simulink model "model"  (R2014a)
settings: Solver=VariableStepAuto  StartTime=0.0  StopTime=10.0  RelTol=1e-3
libraries: powerlib x73
settings Model: Creator=lej  LastModifiedBy=leimhofe
settings DataIOCC: SaveFormat=Dataset
settings OptimizationCC: SimCompilerOptimization=off
settings DebuggingCC: MergeDetectMultiDrivingBlocksExec=error  SolverPrmCheckMsg=none  FrameProcessingCompatibilityMsg=error  AllowSymbolicDim=off
settings HardwareCC: ProdBitPerPointer=64  ProdLargestAtomicFloat=Float  ProdIntDivRoundTo=Zero  ProdEndianess=LittleEndian  ProdWordSize=64  ProdHWDeviceType=Intel->x86-64 (Windows64)
settings RTWCC: RTWCompilerOptimization=off
settings GRTTargetCC: GeneratePreprocessorConditionals=Use local settings
settings ConfigComp: CovMetricSettings=dw  CovHtmlReporting=on  CovSaveCumulativeToWorkspaceVar=on  CovSaveSingleToWorkspaceVar=on  CovExternalEMLEnable=off

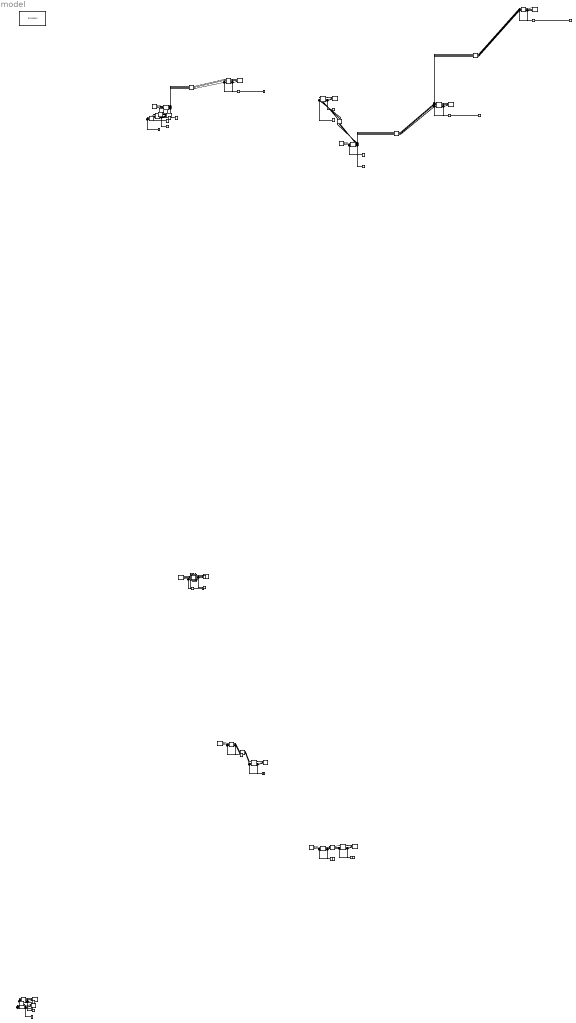
== system model ==
  note: 220000 Volts Power Line
  G_329137671_Termoeléctrica_Cospique : powerlib/Electrical Sources/Three-Phase Source  Voltage=220000  PhaseAngle=0  Frequency=60  InternalConnection=Yg  SpecifyImpedance=on  Resistance=0.8929  Inductance=16.58e-3  ShortCircuitLevel=100e6  BaseVoltage=220000  XRratio=7  BusType=swing  Pref=0  Qref=0  Qmin=-inf  Qmax=inf
  L_{42527718,88597989,108961999,133889140,169000716,169248620,235350409,265884598..265884599,329111639,329112852,329137670,329323507,330857322,331119341} (15 alike) : powerlib/Elements/Three-Phase Series RLC Load  LConnTagsString=A|B|C  Configuration=Y (grounded)  NominalVoltage=220000  NominalFrequency=60  ActivePower=100000  InductivePower=100  CapacitivePower=100  Measurements=None  LoadType=constant Z
  T_108961999__ : powerlib/Elements/Three-Phase Transformer (Two Windings)  Winding1Connection=Yg  UNITS=pu  NominalPower=[ 250e6 , 60 ]  Winding1=[220000,0.002,0.08]  Winding2Connection=Yg  Winding2=[220000,0.002,0.08]  SetSaturation=off  Rm=500  Lm=500  Saturation=[ 0,0 ; 0.0024,1.2 ; 1.0,1.52 ]  Hysteresis=off  DataFile='hysteresis'  SetInitialFlux=off  InitialFluxes=[ 0.8 , -0.8 , 0.7 ]  Measurements=None  MoreParameters=off  BreakLoop=off  DataType=off  TransfoNumber=1
  T_133889140__Ternera : powerlib/Elements/Three-Phase Transformer (Two Windings)  Winding1Connection=Yg  UNITS=pu  NominalPower=[ 250e6 , 60 ]  Winding1=[220000,0.002,0.08]  Winding2Connection=Yg  Winding2=[220000,0.002,0.08]  SetSaturation=off  Rm=500  Lm=500  Saturation=[ 0,0 ; 0.0024,1.2 ; 1.0,1.52 ]  Hysteresis=off  DataFile='hysteresis'  SetInitialFlux=off  InitialFluxes=[ 0.8 , -0.8 , 0.7 ]  Measurements=None  MoreParameters=off  BreakLoop=off  DataType=off  TransfoNumber=1
  T_169000716__ : powerlib/Elements/Three-Phase Transformer (Two Windings)  Winding1Connection=Yg  UNITS=pu  NominalPower=[ 250e6 , 60 ]  Winding1=[220000,0.002,0.08]  Winding2Connection=Yg  Winding2=[220000,0.002,0.08]  SetSaturation=off  Rm=500  Lm=500  Saturation=[ 0,0 ; 0.0024,1.2 ; 1.0,1.52 ]  Hysteresis=off  DataFile='hysteresis'  SetInitialFlux=off  InitialFluxes=[ 0.8 , -0.8 , 0.7 ]  Measurements=None  MoreParameters=off  BreakLoop=off  DataType=off  TransfoNumber=1
  T_169248620_220000_ : powerlib/Elements/Three-Phase Transformer (Two Windings)  Winding1Connection=Yg  UNITS=pu  NominalPower=[ 250e6 , 60 ]  Winding1=[220000,0.002,0.08]  Winding2Connection=Yg  Winding2=[220000,0.002,0.08]  SetSaturation=off  Rm=500  Lm=500  Saturation=[ 0,0 ; 0.0024,1.2 ; 1.0,1.52 ]  Hysteresis=off  DataFile='hysteresis'  SetInitialFlux=off  InitialFluxes=[ 0.8 , -0.8 , 0.7 ]  Measurements=None  MoreParameters=off  BreakLoop=off  DataType=off  TransfoNumber=1
  T_235350409__ : powerlib/Elements/Three-Phase Transformer (Two Windings)  Winding1Connection=Yg  UNITS=pu  NominalPower=[ 250e6 , 60 ]  Winding1=[220000,0.002,0.08]  Winding2Connection=Yg  Winding2=[220000,0.002,0.08]  SetSaturation=off  Rm=500  Lm=500  Saturation=[ 0,0 ; 0.0024,1.2 ; 1.0,1.52 ]  Hysteresis=off  DataFile='hysteresis'  SetInitialFlux=off  InitialFluxes=[ 0.8 , -0.8 , 0.7 ]  Measurements=None  MoreParameters=off  BreakLoop=off  DataType=off  TransfoNumber=1
  T_265884598__ : powerlib/Elements/Three-Phase Transformer (Two Windings)  Winding1Connection=Yg  UNITS=pu  NominalPower=[ 250e6 , 60 ]  Winding1=[220000,0.002,0.08]  Winding2Connection=Yg  Winding2=[220000,0.002,0.08]  SetSaturation=off  Rm=500  Lm=500  Saturation=[ 0,0 ; 0.0024,1.2 ; 1.0,1.52 ]  Hysteresis=off  DataFile='hysteresis'  SetInitialFlux=off  InitialFluxes=[ 0.8 , -0.8 , 0.7 ]  Measurements=None  MoreParameters=off  BreakLoop=off  DataType=off  TransfoNumber=1
  T_265884599__ : powerlib/Elements/Three-Phase Transformer (Two Windings)  Winding1Connection=Yg  UNITS=pu  NominalPower=[ 250e6 , 60 ]  Winding1=[220000,0.002,0.08]  Winding2Connection=Yg  Winding2=[220000,0.002,0.08]  SetSaturation=off  Rm=500  Lm=500  Saturation=[ 0,0 ; 0.0024,1.2 ; 1.0,1.52 ]  Hysteresis=off  DataFile='hysteresis'  SetInitialFlux=off  InitialFluxes=[ 0.8 , -0.8 , 0.7 ]  Measurements=None  MoreParameters=off  BreakLoop=off  DataType=off  TransfoNumber=1
  T_329111639_220000_ : powerlib/Elements/Three-Phase Transformer (Two Windings)  Winding1Connection=Yg  UNITS=pu  NominalPower=[ 250e6 , 60 ]  Winding1=[220000,0.002,0.08]  Winding2Connection=Yg  Winding2=[220000,0.002,0.08]  SetSaturation=off  Rm=500  Lm=500  Saturation=[ 0,0 ; 0.0024,1.2 ; 1.0,1.52 ]  Hysteresis=off  DataFile='hysteresis'  SetInitialFlux=off  InitialFluxes=[ 0.8 , -0.8 , 0.7 ]  Measurements=None  MoreParameters=off  BreakLoop=off  DataType=off  TransfoNumber=1
  T_329112852__ : powerlib/Elements/Three-Phase Transformer (Two Windings)  Winding1Connection=Yg  UNITS=pu  NominalPower=[ 250e6 , 60 ]  Winding1=[220000,0.002,0.08]  Winding2Connection=Yg  Winding2=[220000,0.002,0.08]  SetSaturation=off  Rm=500  Lm=500  Saturation=[ 0,0 ; 0.0024,1.2 ; 1.0,1.52 ]  Hysteresis=off  DataFile='hysteresis'  SetInitialFlux=off  InitialFluxes=[ 0.8 , -0.8 , 0.7 ]  Measurements=None  MoreParameters=off  BreakLoop=off  DataType=off  TransfoNumber=1
  T_329137670__ : powerlib/Elements/Three-Phase Transformer (Two Windings)  Winding1Connection=Yg  UNITS=pu  NominalPower=[ 250e6 , 60 ]  Winding1=[220000,0.002,0.08]  Winding2Connection=Yg  Winding2=[220000,0.002,0.08]  SetSaturation=off  Rm=500  Lm=500  Saturation=[ 0,0 ; 0.0024,1.2 ; 1.0,1.52 ]  Hysteresis=off  DataFile='hysteresis'  SetInitialFlux=off  InitialFluxes=[ 0.8 , -0.8 , 0.7 ]  Measurements=None  MoreParameters=off  BreakLoop=off  DataType=off  TransfoNumber=1
  T_329323507__ : powerlib/Elements/Three-Phase Transformer (Two Windings)  Winding1Connection=Yg  UNITS=pu  NominalPower=[ 250e6 , 60 ]  Winding1=[220000,0.002,0.08]  Winding2Connection=Yg  Winding2=[220000,0.002,0.08]  SetSaturation=off  Rm=500  Lm=500  Saturation=[ 0,0 ; 0.0024,1.2 ; 1.0,1.52 ]  Hysteresis=off  DataFile='hysteresis'  SetInitialFlux=off  InitialFluxes=[ 0.8 , -0.8 , 0.7 ]  Measurements=None  MoreParameters=off  BreakLoop=off  DataType=off  TransfoNumber=1
  T_330857322__ : powerlib/Elements/Three-Phase Transformer (Two Windings)  Winding1Connection=Yg  UNITS=pu  NominalPower=[ 250e6 , 60 ]  Winding1=[220000,0.002,0.08]  Winding2Connection=Yg  Winding2=[220000,0.002,0.08]  SetSaturation=off  Rm=500  Lm=500  Saturation=[ 0,0 ; 0.0024,1.2 ; 1.0,1.52 ]  Hysteresis=off  DataFile='hysteresis'  SetInitialFlux=off  InitialFluxes=[ 0.8 , -0.8 , 0.7 ]  Measurements=None  MoreParameters=off  BreakLoop=off  DataType=off  TransfoNumber=1
  T_331119341__ : powerlib/Elements/Three-Phase Transformer (Two Windings)  Winding1Connection=Yg  UNITS=pu  NominalPower=[ 250e6 , 60 ]  Winding1=[220000,0.002,0.08]  Winding2Connection=Yg  Winding2=[220000,0.002,0.08]  SetSaturation=off  Rm=500  Lm=500  Saturation=[ 0,0 ; 0.0024,1.2 ; 1.0,1.52 ]  Hysteresis=off  DataFile='hysteresis'  SetInitialFlux=off  InitialFluxes=[ 0.8 , -0.8 , 0.7 ]  Measurements=None  MoreParameters=off  BreakLoop=off  DataType=off  TransfoNumber=1
  T_42527718__Central_electrica_Torca : powerlib/Elements/Three-Phase Transformer (Two Windings)  Winding1Connection=Yg  UNITS=pu  NominalPower=[ 250e6 , 60 ]  Winding1=[220000,0.002,0.08]  Winding2Connection=Yg  Winding2=[220000,0.002,0.08]  SetSaturation=off  Rm=500  Lm=500  Saturation=[ 0,0 ; 0.0024,1.2 ; 1.0,1.52 ]  Hysteresis=off  DataFile='hysteresis'  SetInitialFlux=off  InitialFluxes=[ 0.8 , -0.8 , 0.7 ]  Measurements=None  MoreParameters=off  BreakLoop=off  DataType=off  TransfoNumber=1
  T_88597989__Sabanalarga : powerlib/Elements/Three-Phase Transformer (Two Windings)  Winding1Connection=Yg  UNITS=pu  NominalPower=[ 250e6 , 60 ]  Winding1=[220000,0.002,0.08]  Winding2Connection=Yg  Winding2=[220000,0.002,0.08]  SetSaturation=off  Rm=500  Lm=500  Saturation=[ 0,0 ; 0.0024,1.2 ; 1.0,1.52 ]  Hysteresis=off  DataFile='hysteresis'  SetInitialFlux=off  InitialFluxes=[ 0.8 , -0.8 , 0.7 ]  Measurements=None  MoreParameters=off  BreakLoop=off  DataType=off  TransfoNumber=1
  _CN_108961999_220000_CN_133889140_220000 : powerlib/Elements/Distributed Parameters Line  Phases=3  Frequency=60  Resistance=[0.01273 0.3864]  Inductance="[0.9337e-3  4.1264e-3]"  Capacitance=[12.74e-9 7.751e-9]  Length=12.6446  x1=[0 0 0 0; 0.0001244 0 0 0; 0.0002488 0 0 0; 0.0003733 0 0 0; 0.0004977 0 0 0; 0.0006221 0 0 0]  x2=[0 0 0 0; 0.0001244 0 0 0; 0.0002488 0 0 0; 0.0003733 0 0 0; 0.0004977 0 0 0; 0.0006221 0 0 0]  x3=[0 0 0 0; 0.0001244 0 0 0; 0.0002488 0 0 0; 0.0003733 0 0 0; 0.0004977 0 0 0; 0.0006221 0 0 0]  x4=[0 0 0 0; 0.0001244 0 0 0; 0.0002488 0 0 0; 0.0003733 0 0 0; 0.0004977 0 0 0; 0.0006221 0 0 0]  x5=0  V1=ones(3,3)  V2=ones(3,3)  I1=ones(3,3)  I2=ones(3,3)  nHarmo=1  Measurements=None
  _CN_108961999_220000_CN_329137671_220000 : powerlib/Elements/Distributed Parameters Line  Phases=3  Frequency=60  Resistance=[0.01273 0.3864]  Inductance="[0.9337e-3  4.1264e-3]"  Capacitance=[12.74e-9 7.751e-9]  Length=18.2529  x1=[0 0 0 0; 0.0001244 0 0 0; 0.0002488 0 0 0; 0.0003733 0 0 0; 0.0004977 0 0 0; 0.0006221 0 0 0]  x2=[0 0 0 0; 0.0001244 0 0 0; 0.0002488 0 0 0; 0.0003733 0 0 0; 0.0004977 0 0 0; 0.0006221 0 0 0]  x3=[0 0 0 0; 0.0001244 0 0 0; 0.0002488 0 0 0; 0.0003733 0 0 0; 0.0004977 0 0 0; 0.0006221 0 0 0]  x4=[0 0 0 0; 0.0001244 0 0 0; 0.0002488 0 0 0; 0.0003733 0 0 0; 0.0004977 0 0 0; 0.0006221 0 0 0]  x5=0  V1=ones(3,3)  V2=ones(3,3)  I1=ones(3,3)  I2=ones(3,3)  nHarmo=1  Measurements=None
  _CN_108961999_220000_CN_88597989_220000 : powerlib/Elements/Distributed Parameters Line  Phases=3  Frequency=60  Resistance=[0.01273 0.3864]  Inductance="[0.9337e-3  4.1264e-3]"  Capacitance=[12.74e-9 7.751e-9]  Length=72.0533  x1=[0 0 0 0; 0.0001244 0 0 0; 0.0002488 0 0 0; 0.0003733 0 0 0; 0.0004977 0 0 0; 0.0006221 0 0 0]  x2=[0 0 0 0; 0.0001244 0 0 0; 0.0002488 0 0 0; 0.0003733 0 0 0; 0.0004977 0 0 0; 0.0006221 0 0 0]  x3=[0 0 0 0; 0.0001244 0 0 0; 0.0002488 0 0 0; 0.0003733 0 0 0; 0.0004977 0 0 0; 0.0006221 0 0 0]  x4=[0 0 0 0; 0.0001244 0 0 0; 0.0002488 0 0 0; 0.0003733 0 0 0; 0.0004977 0 0 0; 0.0006221 0 0 0]  x5=0  V1=ones(3,3)  V2=ones(3,3)  I1=ones(3,3)  I2=ones(3,3)  nHarmo=1  Measurements=None
  _CN_169000716_220000_CN_169248620_220000 : powerlib/Elements/Distributed Parameters Line  Phases=3  Frequency=60  Resistance=[0.01273 0.3864]  Inductance="[0.9337e-3  4.1264e-3]"  Capacitance=[12.74e-9 7.751e-9]  Length=25.7585  x1=[0 0 0 0; 0.0001244 0 0 0; 0.0002488 0 0 0; 0.0003733 0 0 0; 0.0004977 0 0 0; 0.0006221 0 0 0]  x2=[0 0 0 0; 0.0001244 0 0 0; 0.0002488 0 0 0; 0.0003733 0 0 0; 0.0004977 0 0 0; 0.0006221 0 0 0]  x3=[0 0 0 0; 0.0001244 0 0 0; 0.0002488 0 0 0; 0.0003733 0 0 0; 0.0004977 0 0 0; 0.0006221 0 0 0]  x4=[0 0 0 0; 0.0001244 0 0 0; 0.0002488 0 0 0; 0.0003733 0 0 0; 0.0004977 0 0 0; 0.0006221 0 0 0]  x5=0  V1=ones(3,3)  V2=ones(3,3)  I1=ones(3,3)  I2=ones(3,3)  nHarmo=1  Measurements=None
  _CN_235350409_220000_CN_42527718_220000 : powerlib/Elements/Distributed Parameters Line  Phases=3  Frequency=60  Resistance=[0.01273 0.3864]  Inductance="[0.9337e-3  4.1264e-3]"  Capacitance=[12.74e-9 7.751e-9]  Length=17.8988  x1=[0 0 0 0; 0.0001244 0 0 0; 0.0002488 0 0 0; 0.0003733 0 0 0; 0.0004977 0 0 0; 0.0006221 0 0 0]  x2=[0 0 0 0; 0.0001244 0 0 0; 0.0002488 0 0 0; 0.0003733 0 0 0; 0.0004977 0 0 0; 0.0006221 0 0 0]  x3=[0 0 0 0; 0.0001244 0 0 0; 0.0002488 0 0 0; 0.0003733 0 0 0; 0.0004977 0 0 0; 0.0006221 0 0 0]  x4=[0 0 0 0; 0.0001244 0 0 0; 0.0002488 0 0 0; 0.0003733 0 0 0; 0.0004977 0 0 0; 0.0006221 0 0 0]  x5=0  V1=ones(3,3)  V2=ones(3,3)  I1=ones(3,3)  I2=ones(3,3)  nHarmo=1  Measurements=None
  _CN_265884598_220000_CN_265884599_220000 : powerlib/Elements/Distributed Parameters Line  Phases=3  Frequency=60  Resistance=[0.01273 0.3864]  Inductance="[0.9337e-3  4.1264e-3]"  Capacitance=[12.74e-9 7.751e-9]  Length=2.0739  x1=[0 0 0 0; 0.0001244 0 0 0; 0.0002488 0 0 0; 0.0003733 0 0 0; 0.0004977 0 0 0; 0.0006221 0 0 0]  x2=[0 0 0 0; 0.0001244 0 0 0; 0.0002488 0 0 0; 0.0003733 0 0 0; 0.0004977 0 0 0; 0.0006221 0 0 0]  x3=[0 0 0 0; 0.0001244 0 0 0; 0.0002488 0 0 0; 0.0003733 0 0 0; 0.0004977 0 0 0; 0.0006221 0 0 0]  x4=[0 0 0 0; 0.0001244 0 0 0; 0.0002488 0 0 0; 0.0003733 0 0 0; 0.0004977 0 0 0; 0.0006221 0 0 0]  x5=0  V1=ones(3,3)  V2=ones(3,3)  I1=ones(3,3)  I2=ones(3,3)  nHarmo=1  Measurements=None
  _CN_329112852_220000_CN_329323507_220000 : powerlib/Elements/Distributed Parameters Line  Phases=3  Frequency=60  Resistance=[0.01273 0.3864]  Inductance="[0.9337e-3  4.1264e-3]"  Capacitance=[12.74e-9 7.751e-9]  Length=16.1025  x1=[0 0 0 0; 0.0001244 0 0 0; 0.0002488 0 0 0; 0.0003733 0 0 0; 0.0004977 0 0 0; 0.0006221 0 0 0]  x2=[0 0 0 0; 0.0001244 0 0 0; 0.0002488 0 0 0; 0.0003733 0 0 0; 0.0004977 0 0 0; 0.0006221 0 0 0]  x3=[0 0 0 0; 0.0001244 0 0 0; 0.0002488 0 0 0; 0.0003733 0 0 0; 0.0004977 0 0 0; 0.0006221 0 0 0]  x4=[0 0 0 0; 0.0001244 0 0 0; 0.0002488 0 0 0; 0.0003733 0 0 0; 0.0004977 0 0 0; 0.0006221 0 0 0]  x5=0  V1=ones(3,3)  V2=ones(3,3)  I1=ones(3,3)  I2=ones(3,3)  nHarmo=1  Measurements=None
  _CN_329137670_220000_CN_329111639_220000 : powerlib/Elements/Distributed Parameters Line  Phases=3  Frequency=60  Resistance=[0.01273 0.3864]  Inductance="[0.9337e-3  4.1264e-3]"  Capacitance=[12.74e-9 7.751e-9]  Length=47.1141  x1=[0 0 0 0; 0.0001244 0 0 0; 0.0002488 0 0 0; 0.0003733 0 0 0; 0.0004977 0 0 0; 0.0006221 0 0 0]  x2=[0 0 0 0; 0.0001244 0 0 0; 0.0002488 0 0 0; 0.0003733 0 0 0; 0.0004977 0 0 0; 0.0006221 0 0 0]  x3=[0 0 0 0; 0.0001244 0 0 0; 0.0002488 0 0 0; 0.0003733 0 0 0; 0.0004977 0 0 0; 0.0006221 0 0 0]  x4=[0 0 0 0; 0.0001244 0 0 0; 0.0002488 0 0 0; 0.0003733 0 0 0; 0.0004977 0 0 0; 0.0006221 0 0 0]  x5=0  V1=ones(3,3)  V2=ones(3,3)  I1=ones(3,3)  I2=ones(3,3)  nHarmo=1  Measurements=None
  _CN_329137670_220000_CN_329112852_220000 : powerlib/Elements/Distributed Parameters Line  Phases=3  Frequency=60  Resistance=[0.01273 0.3864]  Inductance="[0.9337e-3  4.1264e-3]"  Capacitance=[12.74e-9 7.751e-9]  Length=90.7454  x1=[0 0 0 0; 0.0001244 0 0 0; 0.0002488 0 0 0; 0.0003733 0 0 0; 0.0004977 0 0 0; 0.0006221 0 0 0]  x2=[0 0 0 0; 0.0001244 0 0 0; 0.0002488 0 0 0; 0.0003733 0 0 0; 0.0004977 0 0 0; 0.0006221 0 0 0]  x3=[0 0 0 0; 0.0001244 0 0 0; 0.0002488 0 0 0; 0.0003733 0 0 0; 0.0004977 0 0 0; 0.0006221 0 0 0]  x4=[0 0 0 0; 0.0001244 0 0 0; 0.0002488 0 0 0; 0.0003733 0 0 0; 0.0004977 0 0 0; 0.0006221 0 0 0]  x5=0  V1=ones(3,3)  V2=ones(3,3)  I1=ones(3,3)  I2=ones(3,3)  nHarmo=1  Measurements=None
  _CN_330857322_220000_CN_331119341_220000 : powerlib/Elements/Distributed Parameters Line  Phases=3  Frequency=60  Resistance=[0.01273 0.3864]  Inductance="[0.9337e-3  4.1264e-3]"  Capacitance=[12.74e-9 7.751e-9]  Length=6.5131  x1=[0 0 0 0; 0.0001244 0 0 0; 0.0002488 0 0 0; 0.0003733 0 0 0; 0.0004977 0 0 0; 0.0006221 0 0 0]  x2=[0 0 0 0; 0.0001244 0 0 0; 0.0002488 0 0 0; 0.0003733 0 0 0; 0.0004977 0 0 0; 0.0006221 0 0 0]  x3=[0 0 0 0; 0.0001244 0 0 0; 0.0002488 0 0 0; 0.0003733 0 0 0; 0.0004977 0 0 0; 0.0006221 0 0 0]  x4=[0 0 0 0; 0.0001244 0 0 0; 0.0002488 0 0 0; 0.0003733 0 0 0; 0.0004977 0 0 0; 0.0006221 0 0 0]  x5=0  V1=ones(3,3)  V2=ones(3,3)  I1=ones(3,3)  I2=ones(3,3)  nHarmo=1  Measurements=None
  bus1 : powerlib/Measurements/Load Flow Bus  LConnTagsString=a  ID=bus1  Vbase=220000  Vref=1  Vangle=0  VLF=1  angleLF=0
      settings: AttributesFormatString=|
      | %<ID>
      | %<Vbase>V
      | %<VLF>pu
      | %<angleLF>deg.
      | %<Name>
  bus10 : powerlib/Measurements/Load Flow Bus  LConnTagsString=a  ID=bus10  Vbase=220000  Vref=1  Vangle=0  VLF=1  angleLF=0
      settings: AttributesFormatString=|
      | %<ID>
      | %<Vbase>V
      | %<VLF>pu
      | %<angleLF>deg.
      | %<Name>
  bus11 : powerlib/Measurements/Load Flow Bus  LConnTagsString=a  ID=bus11  Vbase=220000  Vref=1  Vangle=0  VLF=1  angleLF=0
      settings: AttributesFormatString=|
      | %<ID>
      | %<Vbase>V
      | %<VLF>pu
      | %<angleLF>deg.
      | %<Name>
  bus12 : powerlib/Measurements/Load Flow Bus  LConnTagsString=a  ID=bus12  Vbase=220000  Vref=1  Vangle=0  VLF=1  angleLF=0
      settings: AttributesFormatString=|
      | %<ID>
      | %<Vbase>V
      | %<VLF>pu
      | %<angleLF>deg.
      | %<Name>
  bus13 : powerlib/Measurements/Load Flow Bus  LConnTagsString=a  ID=bus13  Vbase=220000  Vref=1  Vangle=0  VLF=1  angleLF=0
      settings: AttributesFormatString=|
      | %<ID>
      | %<Vbase>V
      | %<VLF>pu
      | %<angleLF>deg.
      | %<Name>
  bus14 : powerlib/Measurements/Load Flow Bus  LConnTagsString=a  ID=bus14  Vbase=220000  Vref=1  Vangle=0  VLF=1  angleLF=0
      settings: AttributesFormatString=|
      | %<ID>
      | %<Vbase>V
      | %<VLF>pu
      | %<angleLF>deg.
      | %<Name>
  bus15 : powerlib/Measurements/Load Flow Bus  LConnTagsString=a  ID=bus15  Vbase=220000  Vref=1  Vangle=0  VLF=1  angleLF=0
      settings: AttributesFormatString=|
      | %<ID>
      | %<Vbase>V
      | %<VLF>pu
      | %<angleLF>deg.
      | %<Name>
  bus16 : powerlib/Measurements/Load Flow Bus  LConnTagsString=a  ID=bus16  Vbase=220000  Vref=1  Vangle=0  VLF=1  angleLF=0
      settings: AttributesFormatString=|
      | %<ID>
      | %<Vbase>V
      | %<VLF>pu
      | %<angleLF>deg.
      | %<Name>
  bus17 : powerlib/Measurements/Load Flow Bus  LConnTagsString=a  ID=bus17  Vbase=220000  Vref=1  Vangle=0  VLF=1  angleLF=0
      settings: AttributesFormatString=|
      | %<ID>
      | %<Vbase>V
      | %<VLF>pu
      | %<angleLF>deg.
      | %<Name>
  bus18 : powerlib/Measurements/Load Flow Bus  LConnTagsString=a  ID=bus18  Vbase=220000  Vref=1  Vangle=0  VLF=1  angleLF=0
      settings: AttributesFormatString=|
      | %<ID>
      | %<Vbase>V
      | %<VLF>pu
      | %<angleLF>deg.
      | %<Name>
  bus19 : powerlib/Measurements/Load Flow Bus  LConnTagsString=a  ID=bus19  Vbase=220000  Vref=1  Vangle=0  VLF=1  angleLF=0
      settings: AttributesFormatString=|
      | %<ID>
      | %<Vbase>V
      | %<VLF>pu
      | %<angleLF>deg.
      | %<Name>
  bus2 : powerlib/Measurements/Load Flow Bus  LConnTagsString=a  ID=bus2  Vbase=220000  Vref=1  Vangle=0  VLF=1  angleLF=0
      settings: AttributesFormatString=|
      | %<ID>
      | %<Vbase>V
      | %<VLF>pu
      | %<angleLF>deg.
      | %<Name>
  bus20 : powerlib/Measurements/Load Flow Bus  LConnTagsString=a  ID=bus20  Vbase=220000  Vref=1  Vangle=0  VLF=1  angleLF=0
      settings: AttributesFormatString=|
      | %<ID>
      | %<Vbase>V
      | %<VLF>pu
      | %<angleLF>deg.
      | %<Name>
  bus21 : powerlib/Measurements/Load Flow Bus  LConnTagsString=a  ID=bus21  Vbase=220000  Vref=1  Vangle=0  VLF=1  angleLF=0
      settings: AttributesFormatString=|
      | %<ID>
      | %<Vbase>V
      | %<VLF>pu
      | %<angleLF>deg.
      | %<Name>
  bus22 : powerlib/Measurements/Load Flow Bus  LConnTagsString=a  ID=bus22  Vbase=220000  Vref=1  Vangle=0  VLF=1  angleLF=0
      settings: AttributesFormatString=|
      | %<ID>
      | %<Vbase>V
      | %<VLF>pu
      | %<angleLF>deg.
      | %<Name>
  bus23 : powerlib/Measurements/Load Flow Bus  LConnTagsString=a  ID=bus23  Vbase=220000  Vref=1  Vangle=0  VLF=1  angleLF=0
      settings: AttributesFormatString=|
      | %<ID>
      | %<Vbase>V
      | %<VLF>pu
      | %<angleLF>deg.
      | %<Name>
  bus24 : powerlib/Measurements/Load Flow Bus  LConnTagsString=a  ID=bus24  Vbase=220000  Vref=1  Vangle=0  VLF=1  angleLF=0
      settings: AttributesFormatString=|
      | %<ID>
      | %<Vbase>V
      | %<VLF>pu
      | %<angleLF>deg.
      | %<Name>
  bus25 : powerlib/Measurements/Load Flow Bus  LConnTagsString=a  ID=bus25  Vbase=220000  Vref=1  Vangle=0  VLF=1  angleLF=0
      settings: AttributesFormatString=|
      | %<ID>
      | %<Vbase>V
      | %<VLF>pu
      | %<angleLF>deg.
      | %<Name>
  bus26 : powerlib/Measurements/Load Flow Bus  LConnTagsString=a  ID=bus26  Vbase=220000  Vref=1  Vangle=0  VLF=1  angleLF=0
      settings: AttributesFormatString=|
      | %<ID>
      | %<Vbase>V
      | %<VLF>pu
      | %<angleLF>deg.
      | %<Name>
  bus27 : powerlib/Measurements/Load Flow Bus  LConnTagsString=a  ID=bus27  Vbase=220000  Vref=1  Vangle=0  VLF=1  angleLF=0
      settings: AttributesFormatString=|
      | %<ID>
      | %<Vbase>V
      | %<VLF>pu
      | %<angleLF>deg.
      | %<Name>
  bus28 : powerlib/Measurements/Load Flow Bus  LConnTagsString=a  ID=bus28  Vbase=220000  Vref=1  Vangle=0  VLF=1  angleLF=0
      settings: AttributesFormatString=|
      | %<ID>
      | %<Vbase>V
      | %<VLF>pu
      | %<angleLF>deg.
      | %<Name>
  bus29 : powerlib/Measurements/Load Flow Bus  LConnTagsString=a  ID=bus29  Vbase=220000  Vref=1  Vangle=0  VLF=1  angleLF=0
      settings: AttributesFormatString=|
      | %<ID>
      | %<Vbase>V
      | %<VLF>pu
      | %<angleLF>deg.
      | %<Name>
  bus3 : powerlib/Measurements/Load Flow Bus  LConnTagsString=a  ID=bus3  Vbase=220000  Vref=1  Vangle=0  VLF=1  angleLF=0
      settings: AttributesFormatString=|
      | %<ID>
      | %<Vbase>V
      | %<VLF>pu
      | %<angleLF>deg.
      | %<Name>
  bus30 : powerlib/Measurements/Load Flow Bus  LConnTagsString=a  ID=bus30  Vbase=220000  Vref=1  Vangle=0  VLF=1  angleLF=0
      settings: AttributesFormatString=|
      | %<ID>
      | %<Vbase>V
      | %<VLF>pu
      | %<angleLF>deg.
      | %<Name>
  bus31 : powerlib/Measurements/Load Flow Bus  LConnTagsString=a  ID=bus31  Vbase=220000  Vref=1  Vangle=0  VLF=1  angleLF=0
      settings: AttributesFormatString=|
      | %<ID>
      | %<Vbase>V
      | %<VLF>pu
      | %<angleLF>deg.
      | %<Name>
  bus4 : powerlib/Measurements/Load Flow Bus  LConnTagsString=a  ID=bus4  Vbase=220000  Vref=1  Vangle=0  VLF=1  angleLF=0
      settings: AttributesFormatString=|
      | %<ID>
      | %<Vbase>V
      | %<VLF>pu
      | %<angleLF>deg.
      | %<Name>
  bus5 : powerlib/Measurements/Load Flow Bus  LConnTagsString=a  ID=bus5  Vbase=220000  Vref=1  Vangle=0  VLF=1  angleLF=0
      settings: AttributesFormatString=|
      | %<ID>
      | %<Vbase>V
      | %<VLF>pu
      | %<angleLF>deg.
      | %<Name>
  bus6 : powerlib/Measurements/Load Flow Bus  LConnTagsString=a  ID=bus6  Vbase=220000  Vref=1  Vangle=0  VLF=1  angleLF=0
      settings: AttributesFormatString=|
      | %<ID>
      | %<Vbase>V
      | %<VLF>pu
      | %<angleLF>deg.
      | %<Name>
  bus7 : powerlib/Measurements/Load Flow Bus  LConnTagsString=a  ID=bus7  Vbase=220000  Vref=1  Vangle=0  VLF=1  angleLF=0
      settings: AttributesFormatString=|
      | %<ID>
      | %<Vbase>V
      | %<VLF>pu
      | %<angleLF>deg.
      | %<Name>
  bus8 : powerlib/Measurements/Load Flow Bus  LConnTagsString=a  ID=bus8  Vbase=220000  Vref=1  Vangle=0  VLF=1  angleLF=0
      settings: AttributesFormatString=|
      | %<ID>
      | %<Vbase>V
      | %<VLF>pu
      | %<angleLF>deg.
      | %<Name>
  bus9 : powerlib/Measurements/Load Flow Bus  LConnTagsString=a  ID=bus9  Vbase=220000  Vref=1  Vangle=0  VLF=1  angleLF=0
      settings: AttributesFormatString=|
      | %<ID>
      | %<Vbase>V
      | %<VLF>pu
      | %<angleLF>deg.
      | %<Name>
  powergui : powerlib/powergui  Priority=1  SimulationMode=Continuous  SolverType=Tustin  SampleTime=50e-6  frequency=60  SPID=off  DisableSnubberDevices=off  DisableRonSwitches=off  DisableVfSwitches=off  SwTol=0  Interpol=off  DisplayEquations=off  Ts=0  methode=off  frequencyindice=60  Pbase=100e6  ErrMax=1e-4  Iterations=50  UnitsV=kV  UnitsW=MW  FunctionMessages=off  echomessages=off  HookPort=off  EnableUseOfTLC=off  x0status=blocks  RestoreLinks=warning  ResistiveCurrentMeasurement=off  Frange=[0:2:500]  Ylog=off  Xlog=on  ShowGrid=off  save=off  variable=ZData  structure=0  ZoomFFT=off  StartTime=0.0  cycles=1  DisplayStyle=1  fundamental=60  FreqAxis=off  MaxFrequency=1000  frequencyindicesteady=1  RmsSteady=1  display=off
  connections:
  _CN_329137670_220000_CN_329111639_220000/LConn1 -- T_329137670__/LConn1 -- _CN_329137670_220000_CN_329112852_220000/LConn1
  _CN_329137670_220000_CN_329111639_220000/LConn2 -- T_329137670__/LConn2 -- _CN_329137670_220000_CN_329112852_220000/LConn2
  _CN_329137670_220000_CN_329111639_220000/LConn3 -- T_329137670__/LConn3 -- _CN_329137670_220000_CN_329112852_220000/LConn3 -- bus1/LConn1
  T_329111639_220000_/LConn1 -- _CN_329137670_220000_CN_329111639_220000/RConn1
  T_329111639_220000_/LConn2 -- _CN_329137670_220000_CN_329111639_220000/RConn2
  _CN_329137670_220000_CN_329111639_220000/RConn3 -- T_329111639_220000_/LConn3 -- bus2/LConn1
  _CN_329137670_220000_CN_329112852_220000/RConn1 -- T_329112852__/LConn1 -- _CN_329112852_220000_CN_329323507_220000/LConn1
  _CN_329137670_220000_CN_329112852_220000/RConn2 -- T_329112852__/LConn2 -- _CN_329112852_220000_CN_329323507_220000/LConn2
  _CN_329137670_220000_CN_329112852_220000/RConn3 -- T_329112852__/LConn3 -- _CN_329112852_220000_CN_329323507_220000/LConn3 -- bus3/LConn1
  T_235350409__/LConn1 -- _CN_235350409_220000_CN_42527718_220000/LConn1
  T_235350409__/LConn2 -- _CN_235350409_220000_CN_42527718_220000/LConn2
  _CN_235350409_220000_CN_42527718_220000/LConn3 -- T_235350409__/LConn3 -- bus4/LConn1
  T_42527718__Central_electrica_Torca/LConn1 -- _CN_235350409_220000_CN_42527718_220000/RConn1
  T_42527718__Central_electrica_Torca/LConn2 -- _CN_235350409_220000_CN_42527718_220000/RConn2
  _CN_235350409_220000_CN_42527718_220000/RConn3 -- T_42527718__Central_electrica_Torca/LConn3 -- bus5/LConn1
  T_169000716__/LConn1 -- _CN_169000716_220000_CN_169248620_220000/LConn1
  T_169000716__/LConn2 -- _CN_169000716_220000_CN_169248620_220000/LConn2
  _CN_169000716_220000_CN_169248620_220000/LConn3 -- T_169000716__/LConn3 -- bus6/LConn1
  T_169248620_220000_/LConn1 -- _CN_169000716_220000_CN_169248620_220000/RConn1
  T_169248620_220000_/LConn2 -- _CN_169000716_220000_CN_169248620_220000/RConn2
  _CN_169000716_220000_CN_169248620_220000/RConn3 -- T_169248620_220000_/LConn3 -- bus7/LConn1
  T_329323507__/LConn1 -- _CN_329112852_220000_CN_329323507_220000/RConn1
  T_329323507__/LConn2 -- _CN_329112852_220000_CN_329323507_220000/RConn2
  _CN_329112852_220000_CN_329323507_220000/RConn3 -- T_329323507__/LConn3 -- bus8/LConn1
  T_265884598__/LConn1 -- _CN_265884598_220000_CN_265884599_220000/LConn1
  T_265884598__/LConn2 -- _CN_265884598_220000_CN_265884599_220000/LConn2
  _CN_265884598_220000_CN_265884599_220000/LConn3 -- T_265884598__/LConn3 -- bus9/LConn1
  T_265884599__/LConn1 -- _CN_265884598_220000_CN_265884599_220000/RConn1
  T_265884599__/LConn2 -- _CN_265884598_220000_CN_265884599_220000/RConn2
  _CN_265884598_220000_CN_265884599_220000/RConn3 -- T_265884599__/LConn3 -- bus10/LConn1
  _CN_108961999_220000_CN_133889140_220000/LConn1 -- T_108961999__/LConn1 -- _CN_108961999_220000_CN_88597989_220000/LConn1 -- _CN_108961999_220000_CN_329137671_220000/LConn1
  _CN_108961999_220000_CN_133889140_220000/LConn2 -- T_108961999__/LConn2 -- _CN_108961999_220000_CN_88597989_220000/LConn2 -- _CN_108961999_220000_CN_329137671_220000/LConn2
  _CN_108961999_220000_CN_133889140_220000/LConn3 -- T_108961999__/LConn3 -- _CN_108961999_220000_CN_88597989_220000/LConn3 -- _CN_108961999_220000_CN_329137671_220000/LConn3 -- bus11/LConn1
  T_133889140__Ternera/LConn1 -- _CN_108961999_220000_CN_133889140_220000/RConn1
  T_133889140__Ternera/LConn2 -- _CN_108961999_220000_CN_133889140_220000/RConn2
  _CN_108961999_220000_CN_133889140_220000/RConn3 -- T_133889140__Ternera/LConn3 -- bus12/LConn1
  T_88597989__Sabanalarga/LConn1 -- _CN_108961999_220000_CN_88597989_220000/RConn1
  T_88597989__Sabanalarga/LConn2 -- _CN_108961999_220000_CN_88597989_220000/RConn2
  _CN_108961999_220000_CN_88597989_220000/RConn3 -- T_88597989__Sabanalarga/LConn3 -- bus13/LConn1
  G_329137671_Termoeléctrica_Cospique/RConn1 -- _CN_108961999_220000_CN_329137671_220000/RConn1
  G_329137671_Termoeléctrica_Cospique/RConn2 -- _CN_108961999_220000_CN_329137671_220000/RConn2
  _CN_108961999_220000_CN_329137671_220000/RConn3 -- G_329137671_Termoeléctrica_Cospique/RConn3 -- bus14/LConn1
  T_330857322__/LConn1 -- _CN_330857322_220000_CN_331119341_220000/LConn1
  T_330857322__/LConn2 -- _CN_330857322_220000_CN_331119341_220000/LConn2
  _CN_330857322_220000_CN_331119341_220000/LConn3 -- T_330857322__/LConn3 -- bus15/LConn1
  T_331119341__/LConn1 -- _CN_330857322_220000_CN_331119341_220000/RConn1
  T_331119341__/LConn2 -- _CN_330857322_220000_CN_331119341_220000/RConn2
  _CN_330857322_220000_CN_331119341_220000/RConn3 -- T_331119341__/LConn3 -- bus16/LConn1
  T_329137670__/RConn1 -- L_329137670/LConn1
  T_329137670__/RConn2 -- L_329137670/LConn2
  L_329137670/LConn3 -- T_329137670__/RConn3 -- bus17/LConn1
  T_329111639_220000_/RConn1 -- L_329111639/LConn1
  T_329111639_220000_/RConn2 -- L_329111639/LConn2
  L_329111639/LConn3 -- T_329111639_220000_/RConn3 -- bus18/LConn1
  T_329112852__/RConn1 -- L_329112852/LConn1
  T_329112852__/RConn2 -- L_329112852/LConn2
  L_329112852/LConn3 -- T_329112852__/RConn3 -- bus19/LConn1
  T_235350409__/RConn1 -- L_235350409/LConn1
  T_235350409__/RConn2 -- L_235350409/LConn2
  L_235350409/LConn3 -- T_235350409__/RConn3 -- bus20/LConn1
  T_42527718__Central_electrica_Torca/RConn1 -- L_42527718/LConn1
  T_42527718__Central_electrica_Torca/RConn2 -- L_42527718/LConn2
  L_42527718/LConn3 -- T_42527718__Central_electrica_Torca/RConn3 -- bus21/LConn1
  T_169000716__/RConn1 -- L_169000716/LConn1
  T_169000716__/RConn2 -- L_169000716/LConn2
  L_169000716/LConn3 -- T_169000716__/RConn3 -- bus22/LConn1
  T_169248620_220000_/RConn1 -- L_169248620/LConn1
  T_169248620_220000_/RConn2 -- L_169248620/LConn2
  L_169248620/LConn3 -- T_169248620_220000_/RConn3 -- bus23/LConn1
  T_329323507__/RConn1 -- L_329323507/LConn1
  T_329323507__/RConn2 -- L_329323507/LConn2
  L_329323507/LConn3 -- T_329323507__/RConn3 -- bus24/LConn1
  T_265884598__/RConn1 -- L_265884598/LConn1
  T_265884598__/RConn2 -- L_265884598/LConn2
  L_265884598/LConn3 -- T_265884598__/RConn3 -- bus25/LConn1
  T_265884599__/RConn1 -- L_265884599/LConn1
  T_265884599__/RConn2 -- L_265884599/LConn2
  L_265884599/LConn3 -- T_265884599__/RConn3 -- bus26/LConn1
  T_108961999__/RConn1 -- L_108961999/LConn1
  T_108961999__/RConn2 -- L_108961999/LConn2
  L_108961999/LConn3 -- T_108961999__/RConn3 -- bus27/LConn1
  T_133889140__Ternera/RConn1 -- L_133889140/LConn1
  T_133889140__Ternera/RConn2 -- L_133889140/LConn2
  L_133889140/LConn3 -- T_133889140__Ternera/RConn3 -- bus28/LConn1
  T_88597989__Sabanalarga/RConn1 -- L_88597989/LConn1
  T_88597989__Sabanalarga/RConn2 -- L_88597989/LConn2
  L_88597989/LConn3 -- T_88597989__Sabanalarga/RConn3 -- bus29/LConn1
  T_330857322__/RConn1 -- L_330857322/LConn1
  T_330857322__/RConn2 -- L_330857322/LConn2
  L_330857322/LConn3 -- T_330857322__/RConn3 -- bus30/LConn1
  T_331119341__/RConn1 -- L_331119341/LConn1
  T_331119341__/RConn2 -- L_331119341/LConn2
  L_331119341/LConn3 -- T_331119341__/RConn3 -- bus31/LConn1
